simulink model "mohinhDLH_thuan"  (R2020a)
settings: Solver=VariableStepAuto  StartTime=0.0  StopTime=10.0  RelTol=1e-3
settings Model: Creator=dell  LastModifiedBy=dell

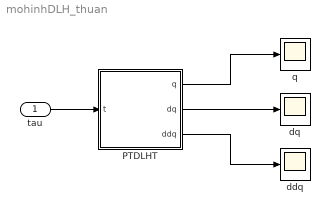
== system mohinhDLH_thuan ==
  tau : Inport
  PTDLHT : MATLAB Function  TreatAsAtomicUnit=on
  ddq : Scope
  dq : Scope
  q : Scope
  wires:
  PTDLHT/1(q) -> q/1
  PTDLHT/2(dq) -> dq/1
  PTDLHT/3(ddq) -> ddq/1
  tau/1 -> PTDLHT/1(t)

== matlab function mohinhDLH_thuan/PTDLHT ==
  data: t input; q output; dq output; ddq output
function [q,dq,ddq] = fcn(t)
